simulink model "FSK_v1"  (R2020b)
settings: Solver=VariableStepAuto  StartTime=0.0  StopTime=30.0  RelTol=1e-3  EnableMultiTasking=on
libraries: dsparch4 x4, commutil2 x2, commchan3 x1, commsink2 x1
settings Model: Creator=Administrator  LastModifiedBy=xiao'xin
settings DataIOCC: LimitDataPoints=on  ReturnWorkspaceOutputs=off
settings OptimizationCC: LifeSpan=inf
settings DebuggingCC: AllowSymbolicDim=off  SFUnexpectedBacktrackingDiag=warning  SFNoUnconditionalDefaultTransitionDiag=warning  SFExecutionAtInitializationDiag=none  ArithmeticOperatorsInVariantConditions=warning
settings ModelReferenceCC: PropagateSignalLabelsOutOfModel=off
settings SFSimCC: SimUseLocalCustomCode=off  CustomCodeUndefinedFunction=UseInterfaceOnly
settings RTWCC: RTWUseLocalCustomCode=off
settings CodeAppCC: StateflowObjectComments=on
settings GRTTargetCC: TargetLangStandard=C89/C90 (ANSI)
settings ConfigComp: CovMetricSettings=dw  CovSaveCumulativeToWorkspaceVar=on  CovSaveSingleToWorkspaceVar=on  CovExternalEMLEnable=off

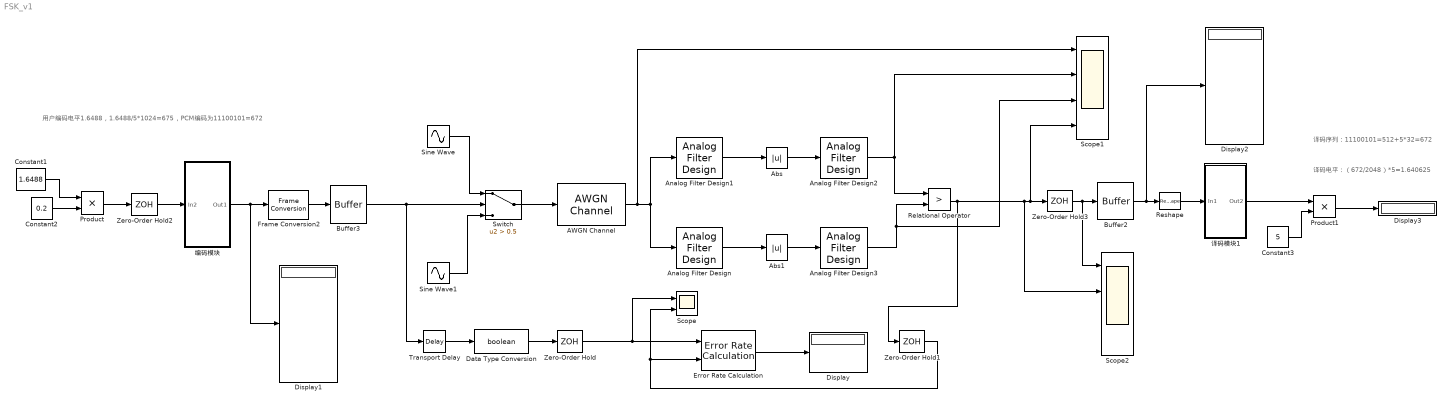
== system FSK_v1 ==
  note: 译码电平：（672/2048）*5=1.640625
  note: 译码序列：11100101=512+5*32=672
  note: 用户编码电平1.6488，1.6488/5*1024=675，PCM编码为11100101=672
  AWGN Channel : commchan3/AWGN Channel  InputProcessing=Columns as channels (frame based)  seed=67  noiseMode="Signal to noise ratio  (SNR)"  EbNodB=0  EsNodB=10  SNRdB=30  bitsPerSym=1  Ps=1  Tsym=1  variance=0.25
  Abs : Abs
  Abs1 : Abs
  Analog Filter Design : dsparch4/Analog Filter Design  method=Butterworth  filttype=Bandpass  N=8  Wlo=80*2*pi  Whi=120*2*pi  Rp=2  Rs=40
  Analog Filter Design1 : dsparch4/Analog Filter Design  method=Butterworth  filttype=Bandpass  N=8  Wlo=180*2*pi  Whi=220*2*pi  Rp=2  Rs=40
  Analog Filter Design2 : dsparch4/Analog Filter Design  method=Butterworth  filttype=Lowpass  N=8  Wlo=180*2*pi  Whi=220*2*pi  Rp=2  Rs=40
  Analog Filter Design3 : dsparch4/Analog Filter Design  method=Butterworth  filttype=Lowpass  N=8  Wlo=80*2*pi  Whi=220*2*pi  Rp=2  Rs=40
  Buffer2 : Buffer  N=8  ic=1  OutputFrames=off
  Buffer3 : Buffer  N=1  OutputFrames=off
  Constant1 : Constant  Value=1.6488
  Constant2 : Constant  Value=0.2
  Constant3 : Constant  Value=5
  Data Type Conversion : DataTypeConversion  OutDataTypeStr=boolean
  Display{,1..3} (4 alike) : Display
  Error Rate Calculation : commsink2/Error Rate Calculation  N=0  st_delay=0  cp_mode=Entire frame  subframe=[]  PMode=Port  WsName=ErrorVec  RsMode2=off  stop=on  numErr=100  maxBits=1e6
  Frame Conversion2 : FrameConversion
  Product : Product
  Product1 : Product
  Relational Operator : RelationalOperator  Operator=>  OutDataTypeStr=boolean  RndMeth=Nearest
  Reshape : Reshape
  Scope : Scope  NumInputPorts=2
  Scope1 : Scope  NumInputPorts=4
  Scope2 : Scope  NumInputPorts=4
  Sine Wave : Sin  Frequency=200*2*pi  SampleTime=0
  Sine Wave1 : Sin  Frequency=100*2*pi  SampleTime=0
  Switch : Switch  Criteria=u2 > Threshold  Threshold=0.5
  Transport Delay : TransportDelay  DelayTime=0.051
  Zero-Order Hold : ZeroOrderHold  SampleTime=0.001
  Zero-Order Hold1 : ZeroOrderHold  SampleTime=0.001
  Zero-Order Hold2 : ZeroOrderHold  SampleTime=9
  Zero-Order Hold3 : ZeroOrderHold  SampleTime=1.17
  编码模块 : Subsystem
  译码模块1 : Subsystem
  wires:
  Sine Wave/1 -> Switch/1
  Sine Wave1/1 -> Switch/3
  Buffer3/1 -> Transport Delay/1, Switch/2
  Switch/1 -> AWGN Channel/1
  Analog Filter Design1/1 -> Abs/1
  AWGN Channel/1 -> Scope1/1, Analog Filter Design/1, Analog Filter Design1/1
  Analog Filter Design/1 -> Abs1/1
  Abs/1 -> Analog Filter Design2/1
  Abs1/1 -> Analog Filter Design3/1
  Analog Filter Design2/1 -> Scope1/2, Relational Operator/1
  Analog Filter Design3/1 -> Scope1/3, Relational Operator/2
  Transport Delay/1 -> Data Type Conversion/1
  Data Type Conversion/1 -> Zero-Order Hold/1
  Error Rate Calculation/1 -> Display/1
  Zero-Order Hold1/1 -> Error Rate Calculation/2, Scope/2
  Zero-Order Hold/1 -> Scope/1, Error Rate Calculation/1
  编码模块/1(Out1) -> Display1/1, Frame Conversion2/1
  Zero-Order Hold2/1 -> 编码模块/1(In2)
  Frame Conversion2/1 -> Buffer3/1
  Product/1 -> Zero-Order Hold2/1
  Constant1/1 -> Product/1
  Constant2/1 -> Product/2
  Relational Operator/1 -> Scope2/2, Scope1/4, Zero-Order Hold3/1, Zero-Order Hold1/1
  Reshape/1 -> 译码模块1/1(In1)
  Buffer2/1 -> Display2/1, Reshape/1
  Zero-Order Hold3/1 -> Scope2/1, Buffer2/1
  Product1/1 -> Display3/1
  译码模块1/1(Out2) -> Product1/1
  Constant3/1 -> Product1/2

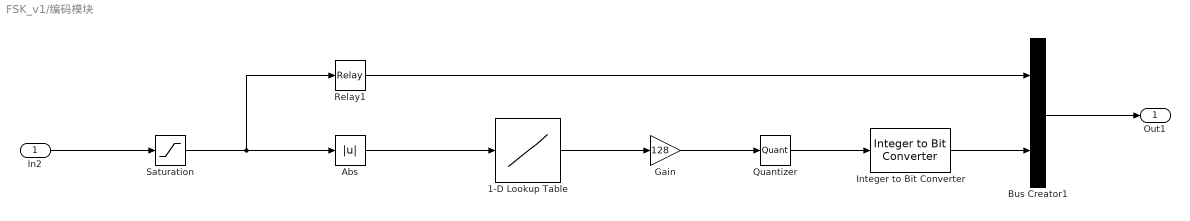
== system FSK_v1/编码模块 ==
  In2 : Inport
  1-D Lookup Table : Lookup_n-D  NumberOfTableDimensions=1  BreakpointsForDimension1=[-1,-1/2,-1/4,-1/8,-1/16,-1/32,-1/64,-1/128,0,1/128,1/64,1/32,1/16,1/8,1/4,1/2,1]  Table=[-1,-7/8,-6/8,-5/8,-4/8,-3/8,-2/8,-1/8,0,1/8,2/8,3/8,4/8,5/8,6/8,7/8,1]  InternalRulePriority=Speed  RndMeth=Simplest  InputSameDT=on
  Abs : Abs
  Bus Creator1 : BusCreator  Inputs=2
  Gain : Gain  Gain=128
  Integer to Bit Converter : commutil2/Integer to Bit Converter  nbits=7  signedInputValues=Unsigned  bitOrder=MSB first  outDtype=Inherit via internal rule
  Quantizer : Quantizer  QuantizationInterval=1
  Relay1 : Relay
  Saturation : Saturate  UpperLimit=1  LowerLimit=-1
  Out1 : Outport
  wires:
  Integer to Bit Converter/1 -> Bus Creator1/2
  Bus Creator1/1 -> Out1/1
  Gain/1 -> Quantizer/1
  In2/1 -> Saturation/1
  1-D Lookup Table/1 -> Gain/1
  Relay1/1 -> Bus Creator1/1
  Quantizer/1 -> Integer to Bit Converter/1
  Abs/1 -> 1-D Lookup Table/1
  Saturation/1 -> Relay1/1, Abs/1

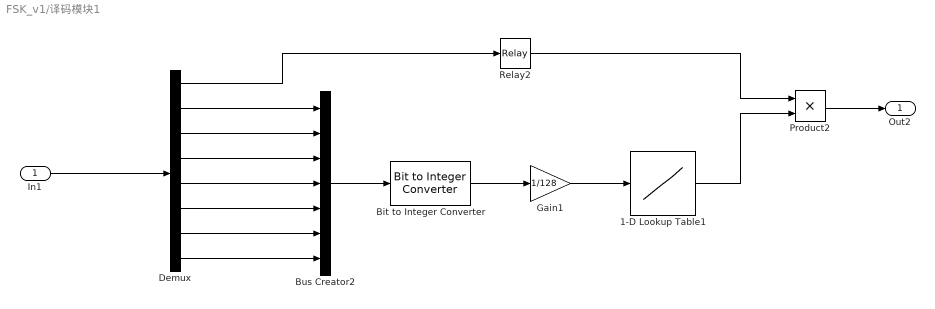
== system FSK_v1/译码模块1 ==
  In1 : Inport
  1-D Lookup Table1 : Lookup_n-D  NumberOfTableDimensions=1  BreakpointsForDimension1=[-1,-7/8,-6/8,-5/8,-4/8,-3/8,-2/8,-1/8,0,1/8,2/8,3/8,4/8,5/8,6/8,7/8,1]  Table=[-1,-1/2,-1/4,-1/8,-1/16,-1/32,-1/64,-1/128,0,1/128,1/64,1/32,1/16,1/8,1/4,1/2,1]  InternalRulePriority=Speed  RndMeth=Simplest  InputSameDT=on
  Bit to Integer Converter : commutil2/Bit to Integer Converter  nbits=7  bitOrder=MSB first  signedOutputValues=Unsigned  outDtype=double  outDtypeSigned=Inherit via internal rule
  Bus Creator2 : BusCreator  Inputs=7
  Demux : Demux  Outputs=8
  Gain1 : Gain  Gain=1/128
  Product2 : Product
  Relay2 : Relay
  Out2 : Outport
  wires:
  Demux/7 -> Bus Creator2/6
  Bit to Integer Converter/1 -> Gain1/1
  Bus Creator2/1 -> Bit to Integer Converter/1
  Product2/1 -> Out2/1
  Demux/5 -> Bus Creator2/4
  Demux/6 -> Bus Creator2/5
  Demux/3 -> Bus Creator2/2
  Demux/4 -> Bus Creator2/3
  1-D Lookup Table1/1 -> Product2/2
  Demux/1 -> Relay2/1
  Gain1/1 -> 1-D Lookup Table1/1
  Demux/8 -> Bus Creator2/7
  Demux/2 -> Bus Creator2/1
  Relay2/1 -> Product2/1
  In1/1 -> Demux/1
